simulink model "linear_dynamic_system"  (R2021a)
settings: Solver=VariableStepAuto  StartTime=0.0  StopTime=1000  RelTol=1e-3
undefined symbols (not defined in the file or in its folder): b, D, g_acc, I, invI, Ix, Iy, Iz, k, Kd_a, Kd_z, Ki_a, Ki_z, Kp_a, Kp_z, L, m, mg
libraries: vrlib x1
settings Model: Creator=filippo  LastModifiedBy=filippo

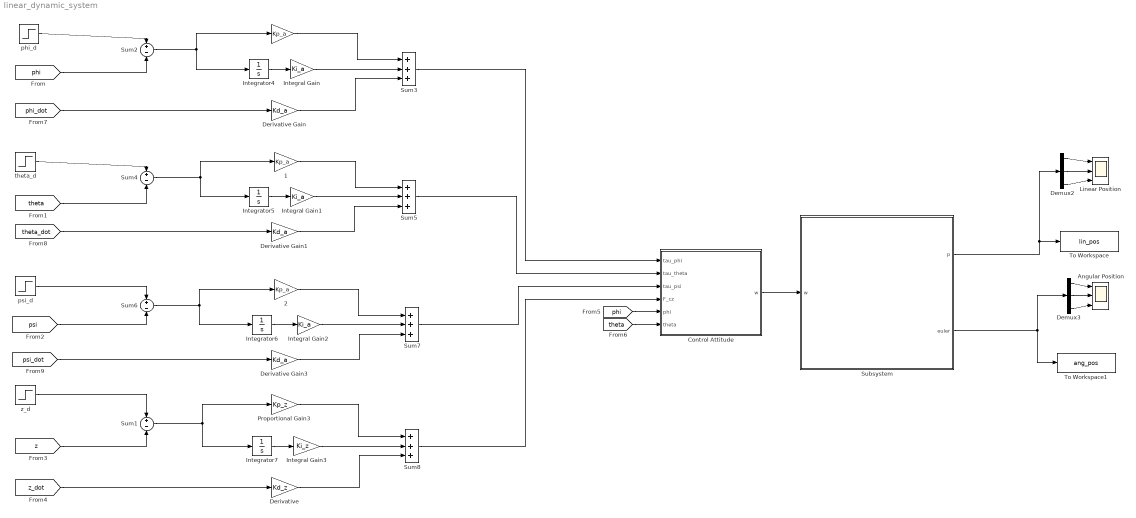
== system linear_dynamic_system ==
  " " : Gain  Gain=Kp_a
  " 1" : Gain  Gain=Kp_a
  " 2" : Gain  Gain=Kp_a
  Angular Position : Scope  NumInputPorts=3
  Control Attitude : MATLAB Function  TreatAsAtomicUnit=on
  Demux2 : Demux  Outputs=3
  Demux3 : Demux  Outputs=3
  "Derivative " : Gain  Gain=Kd_z
  Derivative Gain : Gain  Gain=Kd_a
  Derivative Gain1 : Gain  Gain=Kd_a
  Derivative Gain3 : Gain  Gain=Kd_a
  Integral Gain : Gain  Gain=Ki_a
  Integral Gain1 : Gain  Gain=Ki_a
  Integral Gain2 : Gain  Gain=Ki_a
  Integral Gain3 : Gain  Gain=Ki_z
  Integrator{4..7} (4 alike) : Integrator
  Linear Position : Scope  NumInputPorts=3
  Proportional Gain3 : Gain  Gain=Kp_z
  Subsystem : Subsystem
  Sum{1..2,4,6} (4 alike) : Sum  Inputs=+|-
  Sum{3,5,7..8} (4 alike) : Sum  Inputs=+++
  To Workspace : ToWorkspace  VariableName=lin_pos  SaveFormat=Timeseries  SampleTime=-1
  To Workspace1 : ToWorkspace  VariableName=ang_pos  SaveFormat=Timeseries  SampleTime=-1
  phi_d : Step  After=10  SampleTime=0
  psi_d : Step  After=0  SampleTime=0
  theta_d : Step  After=0  SampleTime=0
  z_d : Step  After=0  SampleTime=0
  wires:
  z_d/1 -> Sum1/1
  " 1"/1 -> Sum5/1
  Proportional Gain3/1 -> Sum8/1
  phi_d/1 -> Sum2/1
  Sum1/1 -> Integrator7/1, Proportional Gain3/1
  Subsystem/2(euler) -> Demux3/1, To Workspace1/1
  theta_d/1 -> Sum4/1
  psi_d/1 -> Sum6/1
  [phi] -> Sum2/2
  Integral Gain2/1 -> Sum7/2
  [theta_dot] -> Derivative Gain1/1
  Sum7/1 -> Control Attitude/3(tau_psi)
  Sum2/1 -> Integrator4/1, " "/1
  Derivative Gain1/1 -> Sum5/3
  "Derivative "/1 -> Sum8/3
  [psi] -> Sum6/2
  Sum3/1 -> Control Attitude/1(tau_phi)
  Demux3/2 -> Angular Position/2
  Integrator4/1 -> Integral Gain/1
  Integral Gain3/1 -> Sum8/2
  [phi_dot] -> Derivative Gain/1
  Derivative Gain/1 -> Sum3/3
  Demux3/3 -> Angular Position/3
  [phi] -> Control Attitude/5(phi)
  Integral Gain1/1 -> Sum5/2
  Demux3/1 -> Angular Position/1
  " "/1 -> Sum3/1
  [theta] -> Control Attitude/6(theta)
  [z_dot] -> "Derivative "/1
  Sum4/1 -> " 1"/1, Integrator5/1
  Derivative Gain3/1 -> Sum7/3
  [psi_dot] -> Derivative Gain3/1
  Demux2/3 -> Linear Position/3
  [theta] -> Sum4/2
  " 2"/1 -> Sum7/1
  Subsystem/1(p) -> Demux2/1, To Workspace/1
  Sum6/1 -> " 2"/1, Integrator6/1
  [z] -> Sum1/2
  Sum8/1 -> Control Attitude/4(F_cz)
  Control Attitude/1(w) -> Subsystem/1(w)
  Integrator6/1 -> Integral Gain2/1
  Integrator7/1 -> Integral Gain3/1
  Integral Gain/1 -> Sum3/2
  Sum5/1 -> Control Attitude/2(tau_theta)
  Integrator5/1 -> Integral Gain1/1
  Demux2/2 -> Linear Position/2
  Demux2/1 -> Linear Position/1

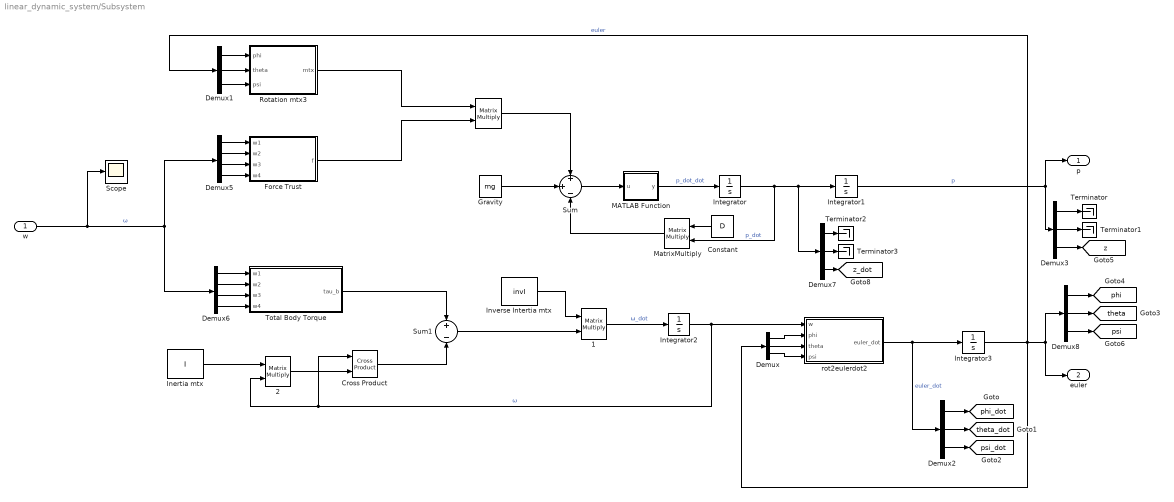
== system linear_dynamic_system/Subsystem ==
  w : Inport
  " " : Product  Multiplication=Matrix(*)
  " 1" : Product  Multiplication=Matrix(*)
  " 2" : Product  Multiplication=Matrix(*)
  Constant : Constant  Value=D
  Cross Product : vrlib/Utilities/Cross Product
  Demux{,1..3,7..8} (6 alike) : Demux  Outputs=3
  Demux5 : Demux
  Demux6 : Demux
  Force Trust : MATLAB Function  TreatAsAtomicUnit=on
  Gravity : Constant  Value=mg  VectorParams1D=off
  Inertia mtx : Constant  Value=I  VectorParams1D=off
  Integrator{,1..3} (4 alike) : Integrator
  Inverse Intertia mtx : Constant  Value=invI
  MATLAB Function : MATLAB Function  TreatAsAtomicUnit=on
  MatrixMultiply : Product  Multiplication=Matrix(*)
  Rotation mtx3 : MATLAB Function  TreatAsAtomicUnit=on
  Scope : Scope
  Sum : Sum  Inputs=+|+|-
  Sum1 : Sum  Inputs=+|-
  Terminator{,1..3} (4 alike) : Terminator
  Total Body Torque : MATLAB Function  TreatAsAtomicUnit=on
  rot2eulerdot2 : MATLAB Function  TreatAsAtomicUnit=on
  p : Outport
  euler : Outport  Port=2
  tag scope: phi=global, phi_dot=global, psi=global, psi_dot=global, theta=global, theta_dot=global, z=global, z_dot=global
  wires:
  Demux3/3 -> [z]
  Demux6/1 -> Total Body Torque/1(w1)
  Demux7/2 -> Terminator3/1
  Demux5/2 -> Force Trust/2(w2)
  Demux8/1 -> [phi]
  Demux6/3 -> Total Body Torque/3(w3)
  Integrator3/1 -> Demux/1, euler/1, Demux8/1, Demux1/1  "euler"
  MatrixMultiply/1 -> Sum/3
  Demux2/1 -> [phi_dot]
  w/1 -> Scope/1, Demux6/1, Demux5/1  "ω"
  Demux6/4 -> Total Body Torque/4(w4)
  Demux2/2 -> [theta_dot]
  Force Trust/1(f) -> " "/2
  Demux1/1 -> Rotation mtx3/1(phi)
  Demux/1 -> rot2eulerdot2/2(phi)
  Demux2/3 -> [psi_dot]
  Demux3/2 -> Terminator1/1
  Demux3/1 -> Terminator/1
  Demux8/3 -> [psi]
  Demux5/1 -> Force Trust/1(w1)
  MATLAB Function/1(y) -> Integrator/1  "p_dot_dot"
  Demux1/2 -> Rotation mtx3/2(theta)
  Demux1/3 -> Rotation mtx3/3(psi)
  " "/1 -> Sum/1
  Constant/1 -> MatrixMultiply/1
  Demux/3 -> rot2eulerdot2/4(psi)
  Inertia mtx/1 -> " 2"/1
  Rotation mtx3/1(mtx) -> " "/1
  rot2eulerdot2/1(euler_dot) -> Integrator3/1, Demux2/1  "euler_dot"
  Demux/2 -> rot2eulerdot2/3(theta)
  Total Body Torque/1(tau_b) -> Sum1/1
  Demux7/3 -> [z_dot]
  Integrator2/1 -> rot2eulerdot2/1(w), Cross Product/1, " 2"/2  "ω"
  Inverse Intertia mtx/1 -> " 1"/1
  Demux7/1 -> Terminator2/1
  Sum1/1 -> " 1"/2
  Sum/1 -> MATLAB Function/1(u)
  " 2"/1 -> Cross Product/2
  Cross Product/1 -> Sum1/2
  " 1"/1 -> Integrator2/1  "ω_dot"
  Demux8/2 -> [theta]
  Demux6/2 -> Total Body Torque/2(w2)
  Integrator/1 -> MatrixMultiply/2, Demux7/1, Integrator1/1  "p_dot"
  Demux5/4 -> Force Trust/4(w4)
  Integrator1/1 -> Demux3/1, p/1  "p"
  Gravity/1 -> Sum/2
  Demux5/3 -> Force Trust/3(w3)

== matlab function linear_dynamic_system/Control Attitude ==
  data: tau_phi input; w output; tau_theta input; tau_psi input; F_cz input; phi input; theta input; Ix parameter; Iy parameter; Iz parameter; L parameter; k parameter; b parameter; m parameter; g_acc parameter
function w = AttitudeControl(tau_phi, tau_theta, tau_psi,F_cz, phi, theta, Ix, Iy, Iz, L, k, b, m, g_acc)
A = [L*k 0 -L*k 0;
     0 L*k 0 -L*k;
     b -b b -b;
     1 1 1 1];
inv_A = inv(A);
U = [-Ix*tau_phi;
     -Iy*tau_theta;
     -Iz*tau_psi;
     m*g_acc/(k*(1-theta)*(1-phi)) + m*F_cz];
w = inv_A*U;
end

== matlab function linear_dynamic_system/Subsystem/Force Trust ==
  data: w1 input; f output [..2]; w2 input; w3 input; w4 input; k parameter; m parameter
function f = F_b(w1,w2,w3,w4,k,m)
mtx = k*[0; 0; w1+w2+w3+w4];
f = mtx;
end

== matlab function linear_dynamic_system/Subsystem/MATLAB Function ==
  data: u input; y output; M parameter
function y = fcn(u, M)
invM = inv(M);
y = invM*u;
end

== matlab function linear_dynamic_system/Subsystem/Total Body Torque ==
  data: w1 input; tau_b output; w2 input; w3 input; w4 input; L parameter; k parameter; b parameter
function tau_b= TotalBodyTorque(w1, w2, w3, w4, L, k, b)
tau_b = [L*k*(w1-w3); L*k*(w2-w4); b*(w1-w2+w3-w4)];
end

== matlab function linear_dynamic_system/Subsystem/rot2eulerdot2 ==
  data: w input; phi input; euler_dot output; theta input; psi input
function euler_dot = rot2euler(w, phi, theta, psi)
R = [1 0 -(theta); 
     0 (1-phi) (1-theta)*(phi);
     0 -(phi) (1-theta)*(1-phi)];
invR = inv(R);
euler_dot = invR*w;
end

== matlab function linear_dynamic_system/Subsystem/Rotation mtx3 ==
  data: phi input; mtx output; theta input; psi input
function mtx = ROTATION(phi, theta, psi)
Rx = [1 0 0; 0 (1-phi) -(phi); 0 (phi) (1-phi)];
Ry = [(1-theta) 0 (theta); 0 1 0; -(theta) 0 (1-theta)];
Rz = [(1-psi) -(psi) 0; (psi) (1-psi) 0; 0 0 1];

% Rot matrix Body-fixed frame wrt Inertial frame
R = Rz * Ry * Rx;
mtx = R;
end
